simulink model "test_rotary_encs_impairments"  (R2025b)
settings: Solver=VariableStepAuto  StartTime=0.0  StopTime=2  RelTol=1e-3
model workspace (MAT data in the model file):
  Ts = Simulink.Parameter
  Ts.Value = 0.001
  Ts.Complexity = 'real'
  Ts.Dimensions = [1 1]
  Ts.Description = 'Sample time.'
  Ts.DataType = 'auto'
  Ts.DocUnits = 's'
libraries: simulink x1, arsenal x1
settings Model: Creator=upattacini  LastModifiedBy=upattacini
settings DataIOCC: SaveOutput=off  DSMLogging=off  SaveTime=off  ReturnWorkspaceOutputs=off

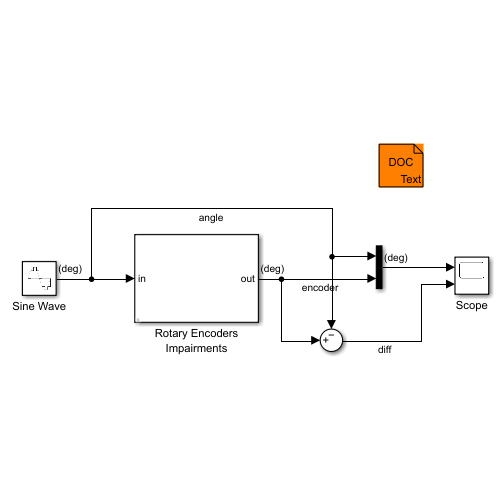
[thumbnail: Simulink's stored preview of the top-level diagram]
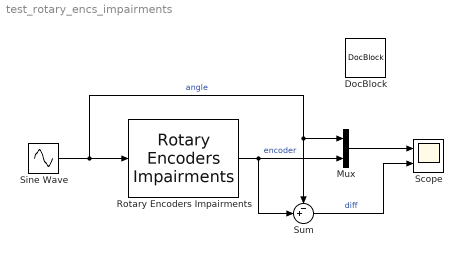
== system test_rotary_encs_impairments ==
  DocBlock : simulink/Model-Wide Utilities/DocBlock  DocumentType=Text
      content=|
      | Rotary Encoders Impairments
      | ===========================
      |
      | - The block simulates the impairments underlying the rotary encoders readouts.
      | - In particular, the block simulates the effects of quantization and noise.
      | - The block enforces the input and output signals units as degrees.
  Mux : Mux  Inputs=2
  Rotary Encoders Impairments : arsenal/Sensing/Rotary Encoders Impairments  bit_resolution=12  bit_noise=4  seed=0  Ts=0.001
  Scope : Scope  NumInputPorts=2
      settings: SampleTime=Ts  ActiveDisplayYMinimum=-63.53317  ActiveDisplayYMaximum=64.03567
  Sine Wave : Sin  Amplitude=50  Frequency=2*pi*0.5  SampleTime=Ts
  Sum : Sum  Inputs=-+|
  wires:
  Mux/1 -> Scope/1
  Sine Wave/1 -> Sum/1, Mux/1, Rotary Encoders Impairments/1  "angle"
  Rotary Encoders Impairments/1 -> Sum/2, Mux/2  "encoder"
  Sum/1 -> Scope/2  "diff"
